simulink model "SafetyCriticalLQR"  (R2020b)
settings: Solver=VariableStepAuto  StartTime=0.0  StopTime=tf_upperbound  RelTol=1e-7
PreLoadFcn:
  | SafetyCriticalLQRParams
values from neighbouring files (symbols this model uses):
  A = [     0 0 1 0;     0 0 0 1;     0 0 0 0;     0 0 0 0 ... (first row only)    [SafetyCriticalLQRParams.m]
  B = [0 0;0 0;1 0;0 1]    [SafetyCriticalLQRParams.m]
  C = eye(4)    [SafetyCriticalLQRParams.m]
  cT = [-2,-2.5]    [SafetyCriticalLQRParams.m]
  D = zeros(4,2)    [SafetyCriticalLQRParams.m]
  Delta = blkdiag(SISODeltaSample,SISODeltaSample)    [ECBFExampleMonteCarloUncertainty.m]    (also in SafetyCriticalLQRParams.m = ss(0,zeros(1,2),zeros(2,1),zeros(2)))
  filterCase = 2    [ECBFExampleMonteCarloUncertainty.m]    (also in SafetyCriticalLQRParams.m = 1)
  gamma = 1    [SafetyCriticalLQRParams.m]
  Ref = [0;0;0;0]    [SafetyCriticalLQRParams.m]
  rT = 1.5    [SafetyCriticalLQRParams.m]
  x0 = [-5;-5;0;0]    [SafetyCriticalLQRParams.m]
undefined symbols (not defined in the file or in its folder): K, P
libraries: simulink x1
settings Model: Creator=Jyot Buch  LastModifiedBy=Jyot Buch

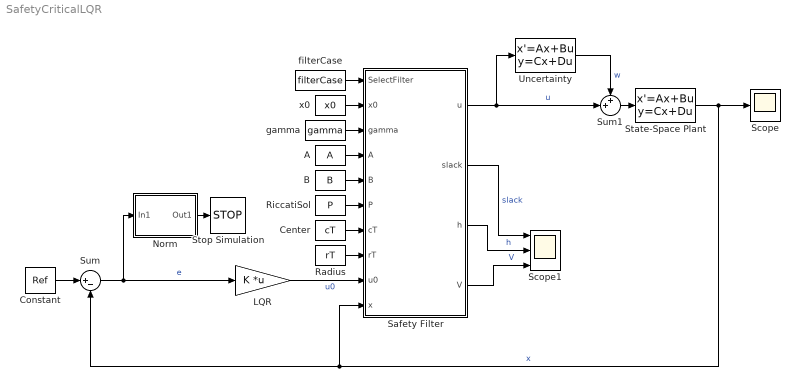
== system SafetyCriticalLQR ==
  A : Constant  Value=A
  B : Constant  Value=B
  Center : Constant  Value=cT
  Constant : Constant  Value=Ref
  LQR : Gain  Gain=K  Multiplication=Matrix(K*u) (u vector)
  Norm : Subsystem
  Radius : Constant  Value=rT
  RiccatiSol : Constant  Value=P
  Safety Filter : MATLAB Function  TreatAsAtomicUnit=on
  Scope : Scope
  Scope1 : Scope  NumInputPorts=3
  State-Space Plant : StateSpace  A=A  B=B  C=C  D=D  InitialCondition=x0
  Stop Simulation : Stop
  Sum : Sum  Inputs=|+-
  Sum1 : Sum  Inputs=++|
  Uncertainty : StateSpace  A=Delta.A  B=Delta.B  C=Delta.C  D=Delta.D  InitialCondition=0
  filterCase : Constant  Value=filterCase
  gamma : Constant  Value=gamma
  x0 : Constant  Value=x0
  wires:
  State-Space Plant/1 -> Safety Filter/10(x), Sum/2, Scope/1  "x"
  Constant/1 -> Sum/1
  Sum/1 -> LQR/1, Norm/1(In1)  "e"
  LQR/1 -> Safety Filter/9(u0)  "u0"
  Safety Filter/1(u) -> Uncertainty/1, Sum1/2  "u"
  Radius/1 -> Safety Filter/8(rT)
  filterCase/1 -> Safety Filter/1(SelectFilter)
  Center/1 -> Safety Filter/7(cT)
  RiccatiSol/1 -> Safety Filter/6(P)
  Safety Filter/3(h) -> Scope1/2  "h"
  Safety Filter/4(V) -> Scope1/3  "V"
  Norm/1(Out1) -> Stop Simulation/1
  x0/1 -> Safety Filter/2(x0)
  gamma/1 -> Safety Filter/3(gamma)
  Safety Filter/2(slack) -> Scope1/1  "slack"
  A/1 -> Safety Filter/4(A)
  B/1 -> Safety Filter/5(B)
  Sum1/1 -> State-Space Plant/1
  Uncertainty/1 -> Sum1/1  "w"

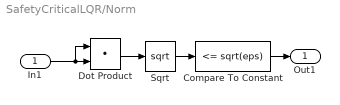
== system SafetyCriticalLQR/Norm ==
  In1 : Inport
  Compare To Constant : simulink/Logic and Bit Operations/Compare To Constant  relop=<=  const=sqrt(eps)  OutDataTypeStr=boolean
  Dot Product : DotProduct  InputSameDT=on  OutDataTypeStr=Inherit: Inherit via internal rule
  Sqrt : Sqrt  SaturateOnIntegerOverflow=on
  Out1 : Outport
  wires:
  In1/1 -> Dot Product/1, Dot Product/2
  Dot Product/1 -> Sqrt/1
  Sqrt/1 -> Compare To Constant/1
  Compare To Constant/1 -> Out1/1

== matlab function SafetyCriticalLQR/Safety Filter ==
  data: SelectFilter input; x0 input; gamma input; A input; B input; P input; cT input; rT input; u0 input; u output; slack output; x input; h output; V output
function [u,slack,h,V] = fcn(SelectFilter,x0,gamma,A,B,P,cT,rT,u0,x)

% Compute h and V
h = (x(1)-cT(1))^2 + (x(2)-cT(2))^2 - rT^2;
V = x'*P*x;
slack = 0;

% Select filter based on the specified case
switch SelectFilter
    case 1
        % Nominal LQR
        u = u0;
                
    case 2
        % CLF-CBF
        [u,slack] = CLFECBFQP(x0,gamma,h,V,A,B,P,cT,x);
        
    otherwise
        % Openloop
        u = u0*0;
end
end

%% CLFCBFQP
function [u,slack] = CLFECBFQP(x0,gamma,h,V,A,B,P,cT,x) %#ok<INUSL>
% This function solves the CLF-ECBF QP at each point integration step.

% Barrier function
hdot = 2*(x(1)-cT(1))*x(3) + 2*(x(2)-cT(2))*x(4);

% Penalty on slack variable
m = 1;

% Design parameters for ECBF
% The first pole should satisfy p1 >= -hdot(x0)/h(x0) -- Since initial
% conditions x(3) and x(4) are zero, this can be any positive real number.
% The second pole should satisfy p2 >= -(hddot(x0) + p1*hdot(x0))/(hdot(x0) + p1*h(x0))
% This constraint is part of the optimization so you can pick any positive
% real number. Optimization will figure out how to satisfy it.

% PerformPolePlacement = true;
% if PerformPolePlacement
    %p1 = 1;
    %p2 = 2;
    %Kalpha = place([0 1;0 0],[0; 1],[-p1 -p2]);
% else
    % Brute-force choosing of gains
    alpha1 = 0.02;
    alpha2 = 0.3;
    Kalpha = [alpha1 alpha2];
% end

% Equality constraints hddot = mu
% Aeq*[u;mu;delta] = beq
Aeq = [2*(x(1)-cT(1)) 2*(x(2)-cT(2)) -1 0];
beq = -2*x(3)^2 - 2*x(4)^2;

% Inequality Constraints Vdot <= -beta*V
Aineq1 = [2*x'*P*B 0 -1];
bineq1 = -x'*(A'*P + P*A)*x - gamma*V;

% Inequality constraints for mu >= -Kalpha*[h;hdot]
Aineq2 = [zeros(1,2), -1, 0];
bineq2 = Kalpha*[h;hdot];

% Inequality Constraints
% Aineq*[u;mu;delta] <= bineq
Aineq = [Aineq1;Aineq2];
bineq = [bineq1;bineq2];

% Solve QP
H = blkdiag(eye(2),0,m);
f = zeros(4,1);
opt = optimoptions('quadprog','Algorithm','active-set','Display','off');
sol = quadprog(H,f,Aineq,bineq,Aeq,beq,[],[],[0;0;0;0],opt);

% Output xdot
u = sol(1:2);
mu = sol(3);
slack = sol(4);
end
